simulink model "SPWMImproved"  (R2023b)
settings: Solver=FixedStepAuto  StartTime=0.0  StopTime=1/1e3  FixedStep=1e-8  RelTol=1e-3
InitFcn:
  | fsw=400e3;
  | ma=0.6;
  | ffund=10e3;
libraries: spsFourierLib x1
settings Model: Creator=enesa  LastModifiedBy=enesa

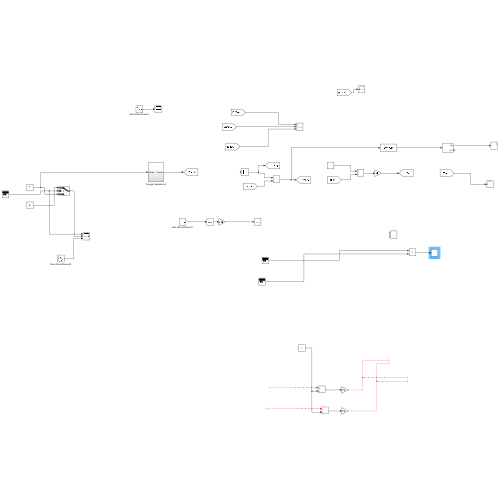
[thumbnail: Simulink's stored preview of the top-level diagram]
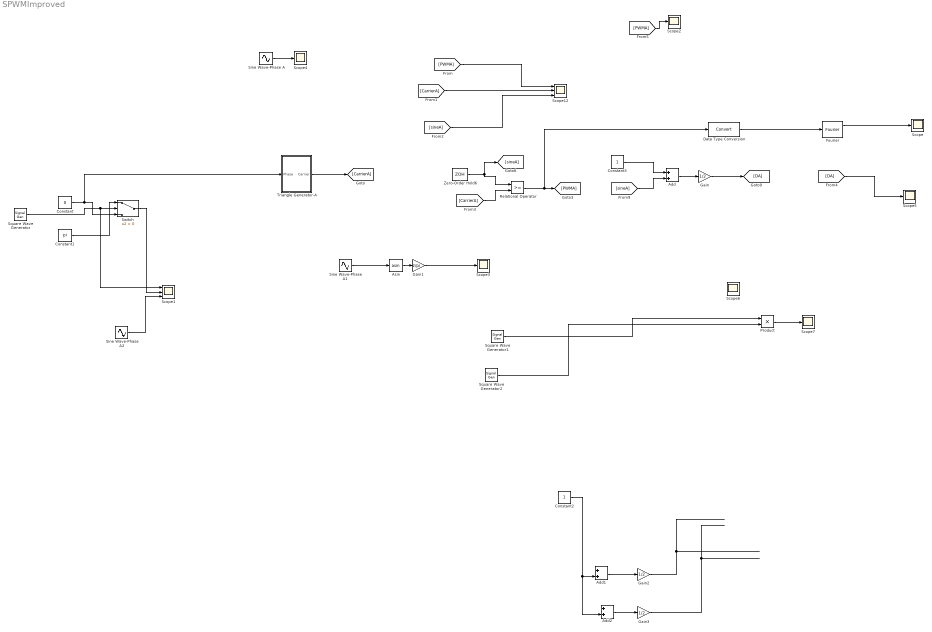
== system SPWMImproved ==
  Add : Sum
  Add1 : Sum
  Add2 : Sum
  Asin : Trigonometry  Operator=asin
  Constant : Constant  Value=0
  Constant1 : Constant  Value=pi
  Constant2 : Constant
  Constant3 : Constant
  Data Type Conversion : DataTypeConversion  SaturateOnIntegerOverflow=off  RndMeth=Floor
  Fourier : spsFourierLib/Fourier  Freq=fsw  n=1  InInit=[0, 0]  Ts=0
  Gain : Gain  Gain=1/2
  Gain1 : Gain  Gain=2/pi
  Gain2 : Gain  Gain=1/2
  Gain3 : Gain  Gain=1/2
  Product : Product
  Relational Operator : RelationalOperator  OutDataTypeStr=boolean  RndMeth=Simplest  InputSameDT=off
  Scope{,2..5,7} (6 alike) : Scope
  Scope1 : Scope  NumInputPorts=3
  Scope12 : Scope  NumInputPorts=3
  Scope6 : Scope  NumInputPorts=2
  Sine Wave-Phase A : Sin  Frequency=2*pi*ffund  SampleTime=0
  Sine Wave-Phase A1 : Sin  Frequency=2*pi*ffund  SampleTime=0
  Sine Wave-Phase A2 : Sin  Frequency=2*pi*ffund  SampleTime=0
  Square Wave Generator : SignalGenerator  WaveForm=square  Frequency=fsw
  Square Wave Generator1 : SignalGenerator  WaveForm=square  Frequency=50e3
  Square Wave Generator2 : SignalGenerator  WaveForm=square  Frequency=20e3
  Switch : Switch  Criteria=u2 > Threshold  SaturateOnIntegerOverflow=off  InputSameDT=off
  Triangle Generator-A : Subsystem
  Zero-Order Hold6 : ZeroOrderHold  SampleTime=1/fsw
  wires:
  Triangle Generator-A/1(Carrier) -> [CarrierA]
  Relational Operator/1 -> Data Type Conversion/1, [PWMA]
  [CarrierA] -> Relational Operator/2
  Constant3/1 -> Add/1
  Gain/1 -> [DA]
  [sineA] -> Add/2
  Add/1 -> Gain/1
  [PWMA] -> Scope12/1
  Sine Wave-Phase A/1 -> Scope4/1
  [CarrierA] -> Scope12/2
  [sineA] -> Scope12/3
  Square Wave Generator/1 -> Scope1/1, Switch/2
  Fourier/1 -> Scope/1
  Data Type Conversion/1 -> Fourier/1
  [PWMA] -> Scope2/1
  Switch/1 -> Scope1/2
  Sine Wave-Phase A1/1 -> Asin/1
  Asin/1 -> Gain1/1
  Zero-Order Hold6/1 -> Relational Operator/1, [sineA]
  Sine Wave-Phase A2/1 -> Scope1/3
  Constant/1 -> Triangle Generator-A/1(Phase), Switch/3
  Constant1/1 -> Switch/1
  Gain1/1 -> Scope3/1
  [DA] -> Scope5/1
  Product/1 -> Scope7/1
  Gain2/1 -> ?
  ? -> Add1/1
  Add2/1 -> Gain3/1
  Constant2/1 -> Add2/2, Add1/2
  Gain3/1 -> ?
  ? -> Add2/1
  Add1/1 -> Gain2/1
  Square Wave Generator1/1 -> Product/1
  Square Wave Generator2/1 -> Product/2

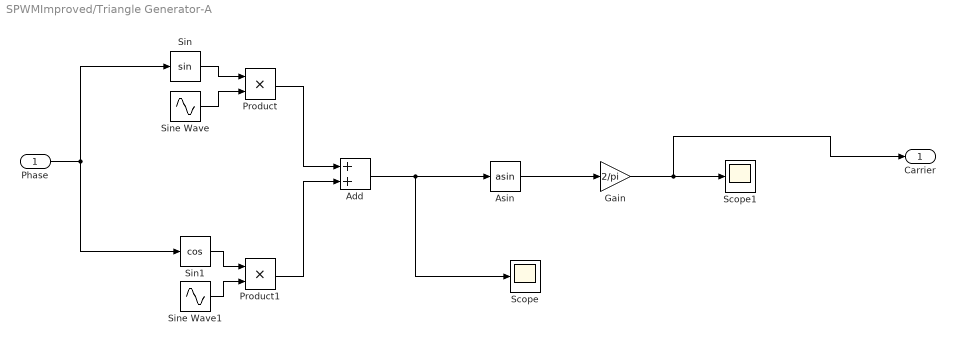
== system SPWMImproved/Triangle Generator-A ==
  Phase : Inport
  Add : Sum
  Asin : Trigonometry  Operator=asin
  Gain : Gain  Gain=2/pi
  Product : Product
  Product1 : Product
  Scope : Scope
  Scope1 : Scope
  Sin : Trigonometry
  Sin1 : Trigonometry  Operator=cos
  Sine Wave : Sin  Frequency=2*pi*fsw  SampleTime=0
  Sine Wave1 : Sin  Frequency=2*pi*fsw  Phase=-pi/2  SampleTime=0
  Carrier : Outport
  wires:
  Sin/1 -> Product/1
  Sine Wave/1 -> Product/2
  Phase/1 -> Sin1/1, Sin/1
  Product/1 -> Add/1
  Asin/1 -> Gain/1
  Gain/1 -> Carrier/1, Scope1/1
  Sine Wave1/1 -> Product1/2
  Product1/1 -> Add/2
  Add/1 -> Asin/1, Scope/1
  Sin1/1 -> Product1/1
